simulink model "q1"  (R2024a)
settings: Solver=VariableStepAuto  StartTime=0.0  StopTime=10.0  RelTol=1e-3
settings Model: Creator=kiani  LastModifiedBy=kiani

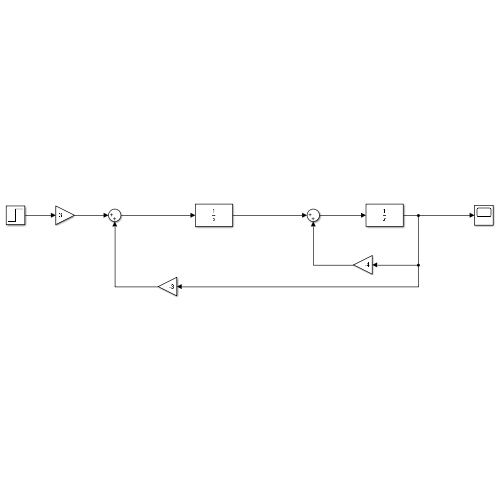
[thumbnail: Simulink's stored preview of the top-level diagram]
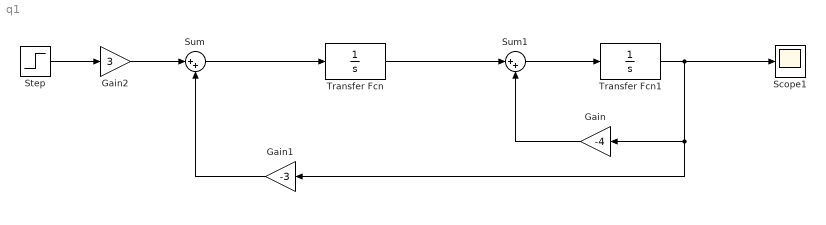
== system q1 ==
  Gain : Gain  Gain=-4
  Gain1 : Gain  Gain=-3
  Gain2 : Gain  Gain=3
  Scope1 : Scope
  Step : Step  Time=0  SampleTime=0
  Sum : Sum  Inputs=|++
  Sum1 : Sum  Inputs=|++
  Transfer Fcn : TransferFcn  Denominator=[1 0]
  Transfer Fcn1 : TransferFcn  Denominator=[1 0]
  wires:
  Sum/1 -> Transfer Fcn/1
  Transfer Fcn/1 -> Sum1/1
  Sum1/1 -> Transfer Fcn1/1
  Gain/1 -> Sum1/2
  Transfer Fcn1/1 -> Scope1/1, Gain1/1, Gain/1
  Gain1/1 -> Sum/2
  Step/1 -> Gain2/1
  Gain2/1 -> Sum/1
